simulink model "bh_3d_pend_sim_CONTROLLED"  (R2021b)
settings: Solver=ode45  StartTime=0.0  StopTime=25  FixedStep=0.001  RelTol=1e-6  AbsTol=1e-6  EnableMultiTasking=on
values from neighbouring files (symbols this model uses):
  K_LAW = [-78.361088012 1.69049101304e-13 6.50451101042e-15 -1.63175637691e-13 78.361088012 1.28612744558e-13 -17.2276366633 -1.91362461096e-14 -9.31673797735e-15 8.02726907722e-14 -17.2276366633 -2.57973956871e-14 ... (39 elements, 3x13)]    [OLD_bh_CONT_DES_RESULTS.mat]    (also in bh_CONT_DES_RESULTS.mat = [-78.361088012 -5.38759787414e-13 -4.00721571005e-14 3.64954)
undefined symbols (not defined in the file or in its folder): DOT_Phi_Theta_Psi, DOT_XYZ, g, Hx, Hy, Hz, Lx, Ly, Lz, M_cart, m_pend, Phi_Theta_Psi, q0_ang_deg, q0_dot_and_deg, sigbuilder_block, X, XYZ, Y, Z
libraries: nesl_utility x14, simulink_extras x11, sm_lib x9
(part 2 of 2)

== matlab function bh_3d_pend_sim_CONTROLLED/MB_PLANT/MB_PLANT/MEAS_ANG/Subsystem1/MATLAB Function ==
  data: bRg input; phi output; theta output; psi output
function [phi, theta, psi] = calc_EUL(bRg)
%#codegen

% bRg = [ ...
%                               cos(phi)*cos(theta),                              cos(theta)*sin(phi),         -sin(theta);
%  cos(phi)*sin(psi)*sin(theta) - cos(psi)*sin(phi), cos(phi)*cos(psi) + sin(phi)*sin(psi)*sin(theta), cos(theta)*sin(psi);
%  sin(phi)*sin(psi) + cos(phi)*cos(psi)*sin(theta), cos(psi)*sin(phi)*sin(theta) - cos(phi)*sin(psi), cos(psi)*cos(theta);
%  ];

phi   = 0; 
theta = 0;
psi   = 0;

theta = -asin(  bRg(1,3) ); % so +/- pi/2 range

phi   = atan2( bRg(1,2) , bRg(1,1)  );  % so +/- pi range
psi   = atan2( bRg(2,3) , bRg(3,3)  );  % so +/- pi range


% THE_TAN_PHI =  bRg(1,2) / bRg(1,1);
% 
% phi   = atan2( THE_TAN_PHI  );  % so +/- pi range
% 
% THE_TAN_PSI =  bRg(2,3) / bRg(3,3);
% 
% psi   = atan2( THE_TAN_PSI  );  % so +/- pi range


% convert to [0 2pi]
% if(phi < 0)   
%     phi = pi + (pi - abs(phi) );   
% end
% 
% if(psi < 0)   
%     psi = pi + (pi - abs(psi) );   
% end

end %function

== matlab function bh_3d_pend_sim_CONTROLLED/MB_PLANT/MB_PLANT/MEAS_ANG/Calc Euler_rates/my_euler_rates ==
  data: theta input; euler_rates output; psi input; p input; q input; r input
function euler_rates = my_euler_rates(theta,psi,p,q,r)
%#codegen

%    This function was generated by the Symbolic Math Toolbox version 7.0.
%    09-Jun-2016 10:28:25

euler_rates = [(r.*cos(psi)+q.*sin(psi))./cos(theta);
                q.*cos(psi)-r.*sin(psi);
               (p.*cos(theta)+r.*cos(psi).*sin(theta)+q.*sin(psi).*sin(theta))./cos(theta)];

== matlab function bh_3d_pend_sim_CONTROLLED/a_circle/MATLAB Function ==
  data: t_clock input; XYZ output; t_to_start input; RADIUS input; ztgt input; w input
function XYZ = fcn(t_clock, t_to_start, RADIUS, ztgt, w)

t    = t_clock - t_to_start;

theta = w*t;

x = RADIUS * cos(theta);
y = RADIUS * sin(theta);
z = ztgt;


XYZ = [x;y;z];
